simulink model "BT8_DieuKhientocdo_PID"  (R2022a)
settings: Solver=FixedStepAuto  StartTime=0.0  StopTime=20  FixedStep=0.01  RelTol=1e-3  EnableMultiTasking=on
libraries: arduinolib x3, arduinosensorlib x1
settings Model: ExtModeTrigDuration=2  Creator=quoc2  LastModifiedBy=kietn
settings OptimizationCC: EnhancedBackFolding=on  PassReuseOutputArgsAs=Individual arguments  ZeroExternalMemoryAtStartup=off  ZeroInternalMemoryAtStartup=off  MaxStackSize=64  OptimizeBlockOrder=speed  DifferentSizesBufferReuse=on  EfficientTunableParamExpr=on
settings DebuggingCC: ParameterTunabilityLossMsg=error
settings HardwareCC: ProdBitPerPointer=32  ProdBitPerSizeT=32  ProdBitPerPtrDiffT=32  ProdLargestAtomicInteger=Long  ProdLargestAtomicFloat=Double  ProdWordSize=32  ProdHWDeviceType=ARM Compatible->ARM Cortex
settings SFSimCC: MATLABDynamicMemAlloc=off
settings RTWCC: SystemTargetFile=ert.tlc  HardwareBoard=ESP32-WROOM(Arduino Compatible)  TLCOptions="-aInlineSetEventsForThisBaseRateFcn=TLC_FALSE -aSuppressMultiTaskScheduler=TLC_FALSE              -aRateBasedStepFcn=0"  TemplateMakefile=ert_default_tmf  Toolchain=ESP32  BuildConfiguration=Faster Runs
settings CodeAppCC: ForceParamTrailComments=on  IgnoreCustomStorageClasses=off  OperatorAnnotations=on  SimulinkDataObjDesc=on  SFDataObjDesc=on  InsertBlockDesc=on
settings ERTTargetCC: SupportContinuousTime=on  SupportVariableSizeSignals=on  ExtMode=on  ExtModeTransport=3  ExtModeStaticAlloc=on  ExtModeStaticAllocSize=65536  ExtModeMexFile=ext_xcp  ExtModeMexArgs=0 3 921600 'E:\Matlab2022a\PID.elf' 3 1000  ExtModeIntrfLevel=Level2 - Open

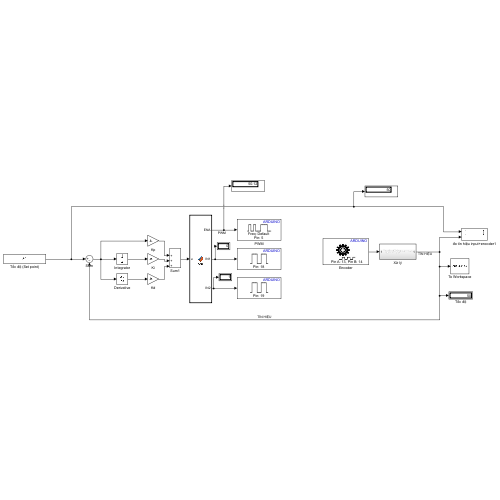
[thumbnail: Simulink's stored preview of the top-level diagram]
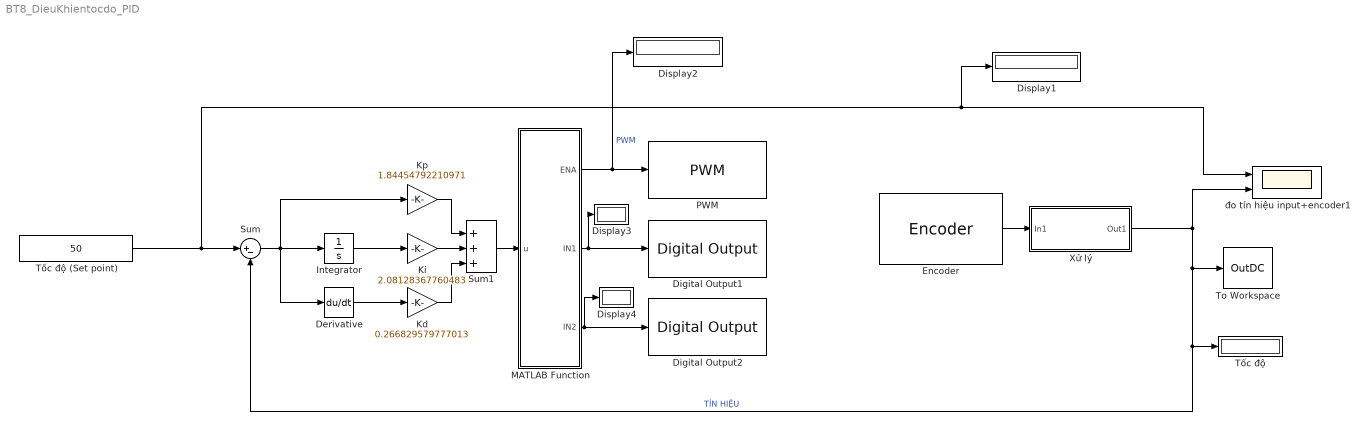
== system BT8_DieuKhientocdo_PID ==
  Derivative : Derivative
  Digital Output1 : arduinolib/Digital Output  pinNumber=18  Direction=output  blockPlatform=arduino
  Digital Output2 : arduinolib/Digital Output  pinNumber=19  Direction=output  blockPlatform=arduino
  Display{1..4} (4 alike) : Display
  Encoder : arduinosensorlib/Encoder  InputA=13  InputB=14  Mode=No reset  SampleTime=-1
      settings: SourceProductBaseCode=ARDUINO
  Integrator : Integrator
  Kd : Gain  Gain=0.266829579777013
  Ki : Gain  Gain=2.08128367760483
  Kp : Gain  Gain=1.84454792210971
  MATLAB Function : MATLAB Function  TreatAsAtomicUnit=on
  PWM : arduinolib/PWM  pinNumber=5  frequencyType=Default  desiredFrequency=490.2  achievableFrequency=490.2
  Sum : Sum  Inputs=|+-
  Sum1 : Sum  Inputs=|+++
  To Workspace : ToWorkspace  VariableName=OutDC  SampleTime=-1
      settings: Save2DSignal=2-D array (concatenate along first dimension)
  Tốc độ : Display
  Tốc độ (Set point) : Constant  Value=50  VectorParams1D=off  OutMin=[-270]  OutMax=[270]  OutDataTypeStr=int16
  Xử lý : Subsystem
  đo tín hiệu input+encoder1 : Scope  NumInputPorts=2
  wires:
  MATLAB Function/1(ENA) -> Display2/1, PWM/1  "PWM"
  Xử lý/1(Out1) -> Tốc độ/1, Sum/2, To Workspace/1, đo tín hiệu input+encoder1/2  "TÍN HIỆU"
  Tốc độ (Set point)/1 -> Display1/1, đo tín hiệu input+encoder1/1, Sum/1
  Sum/1 -> Derivative/1, Integrator/1, Kp/1
  Kp/1 -> Sum1/1
  Encoder/1 -> Xử lý/1(In1)
  Integrator/1 -> Ki/1
  Derivative/1 -> Kd/1
  Ki/1 -> Sum1/2
  Kd/1 -> Sum1/3
  MATLAB Function/2(IN1) -> Display3/1, Digital Output1/1
  MATLAB Function/3(IN2) -> Digital Output2/1, Display4/1
  Sum1/1 -> MATLAB Function/1(u)

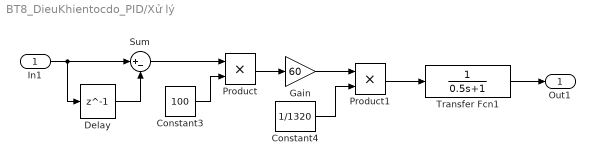
== system BT8_DieuKhientocdo_PID/Xử lý ==
  In1 : Inport
  Constant3 : Constant  Value=100
  Constant4 : Constant  Value=1/1320
  Delay : Delay  DelayLength=1
  Gain : Gain  Gain=60
  Product : Product
  Product1 : Product  OutDataTypeStr=double
  Sum : Sum  Inputs=|+-
  Transfer Fcn1 : TransferFcn  Denominator=[0.5 1]
  Out1 : Outport
  wires:
  Constant4/1 -> Product1/2
  In1/1 -> Sum/1, Delay/1
  Constant3/1 -> Product/2
  Sum/1 -> Product/1
  Delay/1 -> Sum/2
  Gain/1 -> Product1/1
  Product/1 -> Gain/1
  Transfer Fcn1/1 -> Out1/1
  Product1/1 -> Transfer Fcn1/1

== matlab function BT8_DieuKhientocdo_PID/MATLAB Function ==
  data: u input; ENA output; IN1 output; IN2 output
function [ENA,IN1,IN2] = fcn(u)

ENA=abs(u);
if u<0 
    IN1=1; IN2=0;
elseif u>0
    IN1=0; IN2=1;
else 
    IN1=0; IN2=0;
end
